simulink model "Vehicle_Model_2Track_r2018b"  (R2018b)
settings: Solver=FixedStepAuto  SolverName=FixedStepDiscrete  StartTime=T0  StopTime=Tf  FixedStep=Ts  EnableMultiTasking=on
model workspace (MAT data in the model file):
  aKalman = Simulink.Parameter
  aKalman.DataType = 'auto'
  aKalman.Dimensions = [0 0]
  slipEnabler = Simulink.Parameter
  slipEnabler.DataType = 'auto'
  slipEnabler.Dimensions = [0 0]
values from neighbouring files (symbols this model uses):
  longCTRparam = longitController()    [mainVehicleModel_2Track.m]
  pacejkaParam = loadPacejkaParam()    [mainVehicleModel_2Track.m]
  Ts = simulationPars.times.step_size    [mainVehicleModel_2Track.m]
  vehicle_data = getVehicleDataStruct()    [mainVehicleModel_2Track.m]
  X0 = loadInitialConditions    [mainVehicleModel_2Track.m]
undefined symbols (not defined in the file or in its folder): DiscIntNeverNeededParam
libraries: simulink_extras x11
settings Model: Creator=Edoardo  LastModifiedBy=tonegas
settings DataIOCC: LimitDataPoints=on  SaveFormat=Array  ReturnWorkspaceOutputs=on
settings OptimizationCC: DefaultParameterBehavior=Inlined  PassReuseOutputArgsAs=Individual arguments  MaxStackSize=64
settings DebuggingCC: ReadBeforeWriteMsg=DisableAll  WriteAfterWriteMsg=DisableAll  WriteAfterReadMsg=DisableAll  MultiTaskDSMMsg=none  ParameterTunabilityLossMsg=error  SFUnexpectedBacktrackingDiag=warning  SFNoUnconditionalDefaultTransitionDiag=warning  SFExecutionAtInitializationDiag=none
settings HardwareCC: ProdBitPerInt=16  ProdBitPerPointer=16  ProdBitPerSizeT=16  ProdBitPerPtrDiffT=16  ProdLargestAtomicFloat=None  ProdWordSize=16  ProdHWDeviceType=STMicroelectronics->ST10/Super10
settings ModelReferenceCC: UpdateModelReferenceTargets=IfOutOfDate  PropagateSignalLabelsOutOfModel=off
settings SFSimCC: SFSimEcho=off  SimUseLocalCustomCode=off  MATLABDynamicMemAlloc=off
settings RTWCC: SystemTargetFile=ert.tlc  TemplateMakefile=ert_default_tmf  GenerateReport=on  RetainRTWFile=on  RTWUseLocalCustomCode=off  Toolchain=GNU Tools for ARM Embedded Processors  BuildConfiguration=Faster Runs  IncludeHyperlinkInReport=on  LaunchReport=on  GenerateTraceInfo=on  GenerateTraceReport=on  GenerateTraceReportSl=on  GenerateTraceReportSf=on  GenerateTraceReportEml=on
settings CodeAppCC: ForceParamTrailComments=on  IgnoreCustomStorageClasses=off  OperatorAnnotations=on  SimulinkDataObjDesc=on  SFDataObjDesc=on  InsertBlockDesc=on
settings ERTTargetCC: CodeReplacementLibrary=ARM Cortex-M (Optimized)  SupportVariableSizeSignals=on  RootIOFormat=Structure reference  ERTCustomFileTemplate=example_file_process.tlc
settings ConfigComp: CovMetricSettings=dw  CovSaveCumulativeToWorkspaceVar=on  CovSaveSingleToWorkspaceVar=on  CovExternalEMLEnable=off

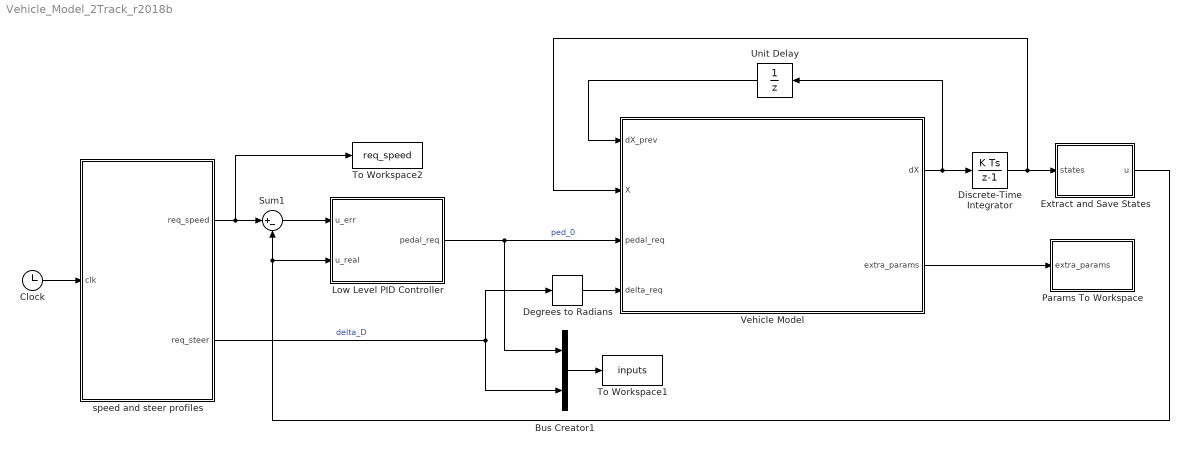
== system Vehicle_Model_2Track_r2018b ==
  Bus Creator1 : BusCreator  Inputs=2
  Clock : Clock
  Degrees to Radians : simulink_extras/Transformations/Degrees to Radians
  Discrete-Time Integrator : DiscreteIntegrator  gainval=1  InitialCondition=X0  SampleTime=-1  ICPrevOutput=DiscIntNeverNeededParam  ICPrevScaledInput=DiscIntNeverNeededParam
  Extract and Save States : Subsystem
  Low Level PID Controller : Subsystem
  Params To Workspace : Subsystem
  Sum1 : Sum  Inputs=|+-
  To Workspace1 : ToWorkspace  VariableName=inputs  SaveFormat=Timeseries  SampleTime=-1
  To Workspace2 : ToWorkspace  VariableName=req_speed  SaveFormat=Timeseries  SampleTime=-1
  Unit Delay : UnitDelay  InitialCondition=zeros(size(X0))  SampleTime=-1  HasFrameUpgradeWarning=on
  Vehicle Model : MATLAB Function  TreatAsAtomicUnit=on
  speed and steer profiles : MATLAB Function  TreatAsAtomicUnit=on
  wires:
  Vehicle Model/2(extra_params) -> Params To Workspace/1(extra_params)
  Discrete-Time Integrator/1 -> Extract and Save States/1(states), Vehicle Model/2(X)
  Vehicle Model/1(dX) -> Unit Delay/1, Discrete-Time Integrator/1
  Bus Creator1/1 -> To Workspace1/1
  speed and steer profiles/2(req_steer) -> Degrees to Radians/1, Bus Creator1/2  "delta_D"
  Degrees to Radians/1 -> Vehicle Model/4(delta_req)
  Clock/1 -> speed and steer profiles/1(clk)
  Low Level PID Controller/1(pedal_req) -> Vehicle Model/3(pedal_req), Bus Creator1/1  "ped_0"
  Unit Delay/1 -> Vehicle Model/1(dX_prev)
  Extract and Save States/1(u) -> Sum1/2, Low Level PID Controller/2(u_real)
  speed and steer profiles/1(req_speed) -> To Workspace2/1, Sum1/1
  Sum1/1 -> Low Level PID Controller/1(u_err)

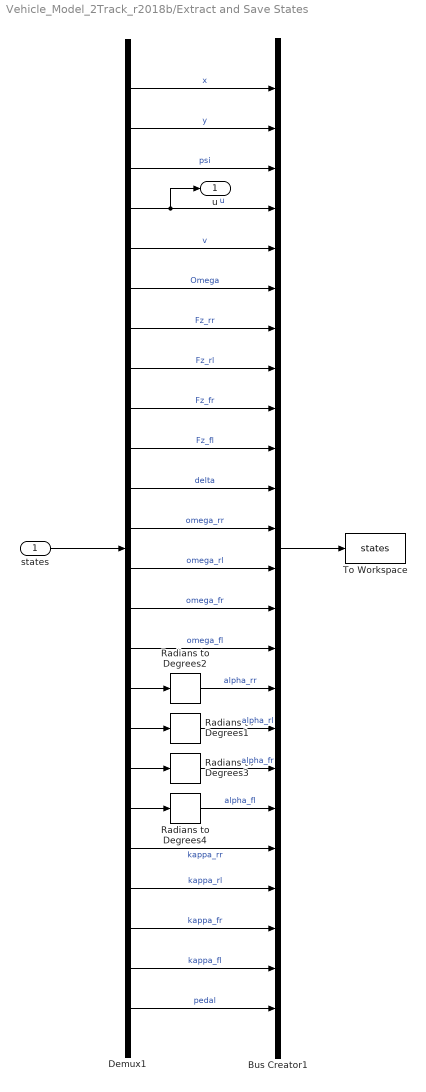
== system Vehicle_Model_2Track_r2018b/Extract and Save States ==
  states : Inport
  Bus Creator1 : BusCreator  Inputs=24
  Demux1 : Demux  Outputs=24
  Radians to Degrees{1..4} (4 alike) : simulink_extras/Transformations/Radians to Degrees
  To Workspace : ToWorkspace  VariableName=states  SaveFormat=Timeseries  SampleTime=-1
  u : Outport
  wires:
  Demux1/13 -> Bus Creator1/13  "omega_rl"
  Demux1/8 -> Bus Creator1/8  "Fz_rl"
  Demux1/23 -> Bus Creator1/23  "kappa_fl"
  Demux1/19 -> Radians to Degrees4/1
  states/1 -> Demux1/1
  Demux1/14 -> Bus Creator1/14  "omega_fr"
  Demux1/7 -> Bus Creator1/7  "Fz_rr"
  Demux1/15 -> Bus Creator1/15  "omega_fl"
  Demux1/3 -> Bus Creator1/3  "psi"
  Demux1/22 -> Bus Creator1/22  "kappa_fr"
  Demux1/4 -> u/1, Bus Creator1/4  "u"
  Demux1/6 -> Bus Creator1/6  "Omega"
  Demux1/11 -> Bus Creator1/11  "delta"
  Demux1/5 -> Bus Creator1/5  "v"
  Demux1/9 -> Bus Creator1/9  "Fz_fr"
  Demux1/21 -> Bus Creator1/21  "kappa_rl"
  Demux1/12 -> Bus Creator1/12  "omega_rr"
  Demux1/17 -> Radians to Degrees1/1
  Demux1/2 -> Bus Creator1/2  "y"
  Demux1/20 -> Bus Creator1/20  "kappa_rr"
  Demux1/10 -> Bus Creator1/10  "Fz_fl"
  Demux1/18 -> Radians to Degrees3/1
  Demux1/1 -> Bus Creator1/1  "x"
  Demux1/16 -> Radians to Degrees2/1
  Bus Creator1/1 -> To Workspace/1
  Radians to Degrees2/1 -> Bus Creator1/16  "alpha_rr"
  Radians to Degrees1/1 -> Bus Creator1/17  "alpha_rl"
  Radians to Degrees3/1 -> Bus Creator1/18  "alpha_fr"
  Radians to Degrees4/1 -> Bus Creator1/19  "alpha_fl"
  Demux1/24 -> Bus Creator1/24  "pedal"

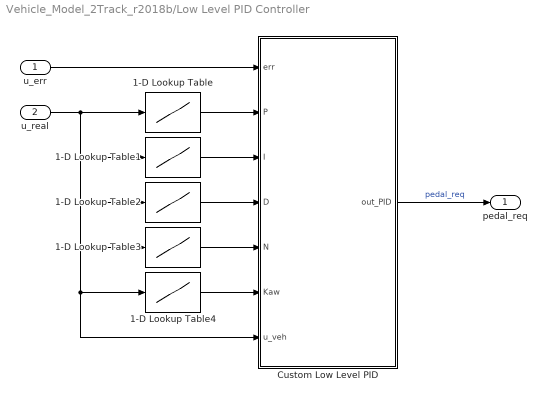
== system Vehicle_Model_2Track_r2018b/Low Level PID Controller ==
  u_err : Inport
  u_real : Inport  Port=2
  1-D Lookup Table : Lookup_n-D  NumberOfTableDimensions=1  BreakpointsForDimension1=longCTRparam.speed_vals_PID_sched  BeginIndexSearchUsingPreviousIndexResult=on  Table=longCTRparam.Kp_vals  ExtrapMethod=Clip  UseLastTableValue=on  InternalRulePriority=Speed  RndMeth=Simplest  InputSameDT=on
  1-D Lookup Table1 : Lookup_n-D  NumberOfTableDimensions=1  BreakpointsForDimension1=longCTRparam.speed_vals_PID_sched  BeginIndexSearchUsingPreviousIndexResult=on  Table=longCTRparam.Ki_vals  ExtrapMethod=Clip  UseLastTableValue=on  InternalRulePriority=Speed  RndMeth=Simplest  InputSameDT=on
  1-D Lookup Table2 : Lookup_n-D  NumberOfTableDimensions=1  BreakpointsForDimension1=longCTRparam.speed_vals_PID_sched  BeginIndexSearchUsingPreviousIndexResult=on  Table=longCTRparam.Kd_vals  ExtrapMethod=Clip  UseLastTableValue=on  InternalRulePriority=Speed  RndMeth=Simplest  InputSameDT=on
  1-D Lookup Table3 : Lookup_n-D  NumberOfTableDimensions=1  BreakpointsForDimension1=longCTRparam.speed_vals_PID_sched  BeginIndexSearchUsingPreviousIndexResult=on  Table=longCTRparam.N_vals  ExtrapMethod=Clip  UseLastTableValue=on  InternalRulePriority=Speed  RndMeth=Simplest  InputSameDT=on
  1-D Lookup Table4 : Lookup_n-D  NumberOfTableDimensions=1  BreakpointsForDimension1=longCTRparam.speed_vals_PID_sched  BeginIndexSearchUsingPreviousIndexResult=on  Table=longCTRparam.Kaw_vals  ExtrapMethod=Clip  UseLastTableValue=on  InternalRulePriority=Speed  RndMeth=Simplest  InputSameDT=on
  Custom Low Level PID : Subsystem
  pedal_req : Outport  VectorParamsAs1DForOutWhenUnconnected=off
  wires:
  1-D Lookup Table/1 -> Custom Low Level PID/2(P)
  u_err/1 -> Custom Low Level PID/1(err)
  u_real/1 -> 1-D Lookup Table4/1, Custom Low Level PID/7(u_veh), 1-D Lookup Table3/1, 1-D Lookup Table2/1, 1-D Lookup Table1/1, 1-D Lookup Table/1
  1-D Lookup Table2/1 -> Custom Low Level PID/4(D)
  1-D Lookup Table3/1 -> Custom Low Level PID/5(N)
  1-D Lookup Table1/1 -> Custom Low Level PID/3(I)
  Custom Low Level PID/1(out_PID) -> pedal_req/1  "pedal_req"
  1-D Lookup Table4/1 -> Custom Low Level PID/6(Kaw)

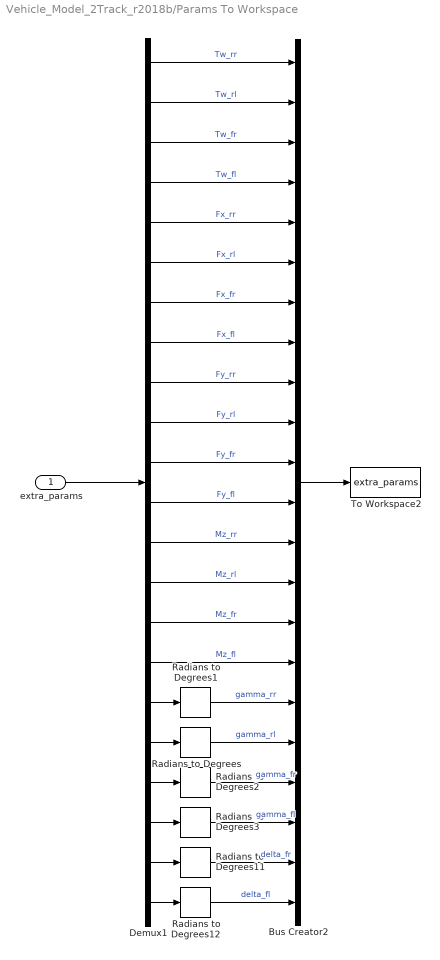
== system Vehicle_Model_2Track_r2018b/Params To Workspace ==
  extra_params : Inport
  Bus Creator2 : BusCreator  Inputs=22
  Demux1 : Demux  Outputs=22
  Radians to Degrees{,1..3,11..12} (6 alike) : simulink_extras/Transformations/Radians to Degrees
  To Workspace2 : ToWorkspace  VariableName=extra_params  SaveFormat=Timeseries  SampleTime=-1
  wires:
  Demux1/17 -> Radians to Degrees1/1
  Demux1/3 -> Bus Creator2/3  "Tw_fr"
  Radians to Degrees3/1 -> Bus Creator2/20  "gamma_fl"
  Demux1/16 -> Bus Creator2/16  "Mz_fl"
  Radians to Degrees1/1 -> Bus Creator2/17  "gamma_rr"
  Radians to Degrees11/1 -> Bus Creator2/21  "delta_fr"
  Demux1/14 -> Bus Creator2/14  "Mz_rl"
  Demux1/4 -> Bus Creator2/4  "Tw_fl"
  Demux1/6 -> Bus Creator2/6  "Fx_rl"
  Demux1/8 -> Bus Creator2/8  "Fx_fl"
  Demux1/13 -> Bus Creator2/13  "Mz_rr"
  Demux1/7 -> Bus Creator2/7  "Fx_fr"
  Demux1/5 -> Bus Creator2/5  "Fx_rr"
  Demux1/9 -> Bus Creator2/9  "Fy_rr"
  Demux1/11 -> Bus Creator2/11  "Fy_fr"
  Demux1/15 -> Bus Creator2/15  "Mz_fr"
  Demux1/10 -> Bus Creator2/10  "Fy_rl"
  Radians to Degrees12/1 -> Bus Creator2/22  "delta_fl"
  Radians to Degrees2/1 -> Bus Creator2/19  "gamma_fr"
  extra_params/1 -> Demux1/1
  Demux1/12 -> Bus Creator2/12  "Fy_fl"
  Bus Creator2/1 -> To Workspace2/1
  Demux1/1 -> Bus Creator2/1  "Tw_rr"
  Demux1/2 -> Bus Creator2/2  "Tw_rl"
  Radians to Degrees/1 -> Bus Creator2/18  "gamma_rl"
  Demux1/18 -> Radians to Degrees/1
  Demux1/19 -> Radians to Degrees2/1
  Demux1/20 -> Radians to Degrees3/1
  Demux1/21 -> Radians to Degrees11/1
  Demux1/22 -> Radians to Degrees12/1

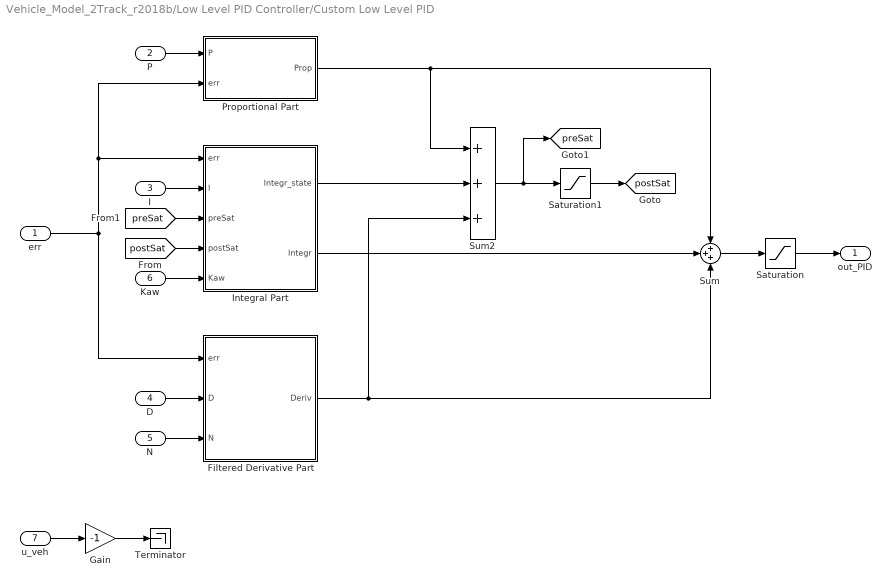
== system Vehicle_Model_2Track_r2018b/Low Level PID Controller/Custom Low Level PID ==
  err : Inport
  P : Inport  Port=2
  I : Inport  Port=3
  D : Inport  Port=4
  N : Inport  Port=5
  Kaw : Inport  Port=6
  u_veh : Inport  Port=7
  Filtered Derivative Part : Subsystem
  Gain : Gain  Gain=-1
  Integral Part : Subsystem
  Proportional Part : Subsystem
  Saturation : Saturate  UpperLimit=1  LowerLimit=-1  LinearizeAsGain=off
  Saturation1 : Saturate  UpperLimit=1  LowerLimit=-1  LinearizeAsGain=off
  Sum : Sum  Inputs=+++
  Sum2 : Sum  Inputs=+++
  Terminator : Terminator
  out_PID : Outport  VectorParamsAs1DForOutWhenUnconnected=off
  tag scope: postSat=global, preSat=global
  wires:
  Sum2/1 -> [preSat], Saturation1/1
  Sum/1 -> Saturation/1
  Saturation/1 -> out_PID/1
  err/1 -> Filtered Derivative Part/1(err), Proportional Part/2(err), Integral Part/1(err)
  Saturation1/1 -> [postSat]
  I/1 -> Integral Part/2(I)
  Integral Part/1(Integr_state) -> Sum2/2
  Integral Part/2(Integr) -> Sum/2
  Proportional Part/1(Prop) -> Sum2/1, Sum/1
  P/1 -> Proportional Part/1(P)
  [preSat] -> Integral Part/3(preSat)
  [postSat] -> Integral Part/4(postSat)
  Filtered Derivative Part/1(Deriv) -> Sum/3, Sum2/3
  D/1 -> Filtered Derivative Part/2(D)
  N/1 -> Filtered Derivative Part/3(N)
  u_veh/1 -> Gain/1
  Gain/1 -> Terminator/1
  Kaw/1 -> Integral Part/5(Kaw)

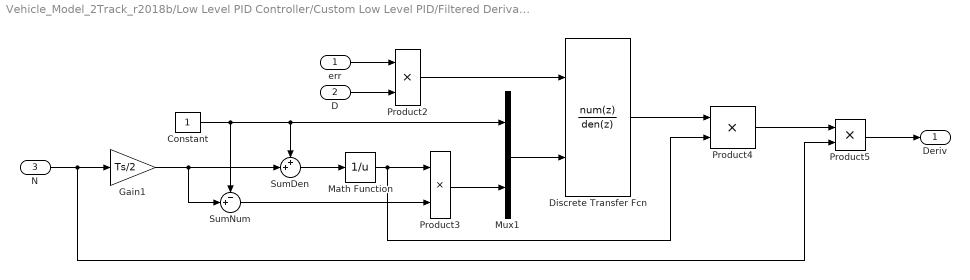
== system Vehicle_Model_2Track_r2018b/Low Level PID Controller/Custom Low Level PID/Filtered Derivative Part ==
  err : Inport
  D : Inport  Port=2
  N : Inport  Port=3
  Constant : Constant
  Discrete Transfer Fcn : DiscreteTransferFcn  Numerator=[1 -1]  DenominatorSource=Input port  SampleTime=Ts  a0EqualsOne=on
      settings: InputPortMap=u0,p3
  Gain1 : Gain  Gain=Ts/2
  Math Function : Math  Operator=reciprocal  SaturateOnIntegerOverflow=on
  Mux1 : Mux  Inputs=2
  Product{2..5} (4 alike) : Product
  SumDen : Sum  Inputs=++|
  SumNum : Sum  Inputs=-+|
  Deriv : Outport  VectorParamsAs1DForOutWhenUnconnected=off
  wires:
  N/1 -> Gain1/1, Product5/2
  Product4/1 -> Product5/1
  SumDen/1 -> Math Function/1
  Math Function/1 -> Product4/2, Product3/1
  SumNum/1 -> Product3/2
  Product2/1 -> Discrete Transfer Fcn/1
  Discrete Transfer Fcn/1 -> Product4/1
  Constant/1 -> SumNum/1, SumDen/1, Mux1/1
  Product3/1 -> Mux1/2
  Mux1/1 -> Discrete Transfer Fcn/2
  Gain1/1 -> SumNum/2, SumDen/2
  err/1 -> Product2/1
  D/1 -> Product2/2
  Product5/1 -> Deriv/1

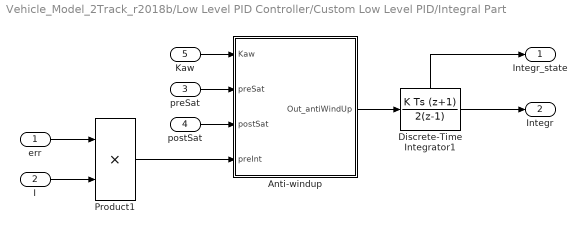
== system Vehicle_Model_2Track_r2018b/Low Level PID Controller/Custom Low Level PID/Integral Part ==
  err : Inport
  I : Inport  Port=2
  preSat : Inport  Port=3
  postSat : Inport  Port=4
  Kaw : Inport  Port=5
  Anti-windup : Subsystem
  Discrete-Time Integrator1 : DiscreteIntegrator  IntegratorMethod=Integration: Trapezoidal  SampleTime=Ts  ShowStatePort=on  ICPrevOutput=DiscIntNeverNeededParam  ICPrevScaledInput=DiscIntNeverNeededParam
  Product1 : Product
  Integr_state : Outport  VectorParamsAs1DForOutWhenUnconnected=off
  Integr : Outport  Port=2  VectorParamsAs1DForOutWhenUnconnected=off
  wires:
  Discrete-Time Integrator1/State -> Integr_state/1
  preSat/1 -> Anti-windup/2(preSat)
  Product1/1 -> Anti-windup/4(preInt)
  postSat/1 -> Anti-windup/3(postSat)
  I/1 -> Product1/2
  Anti-windup/1(Out_antiWindUp) -> Discrete-Time Integrator1/1
  Discrete-Time Integrator1/1 -> Integr/1
  err/1 -> Product1/1
  Kaw/1 -> Anti-windup/1(Kaw)

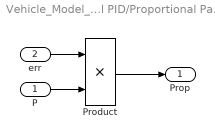
== system Vehicle_Model_2Track_r2018b/Low Level PID Controller/Custom Low Level PID/Proportional Part ==
  P : Inport
  err : Inport  Port=2
  Product : Product
  Prop : Outport  VectorParamsAs1DForOutWhenUnconnected=off
  wires:
  P/1 -> Product/2
  Product/1 -> Prop/1
  err/1 -> Product/1

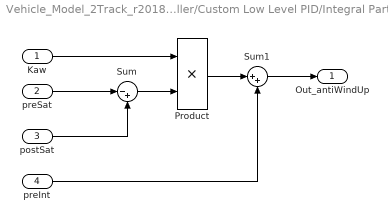
== system Vehicle_Model_2Track_r2018b/Low Level PID Controller/Custom Low Level PID/Integral Part/Anti-windup ==
  Kaw : Inport
  preSat : Inport  Port=2
  postSat : Inport  Port=3
  preInt : Inport  Port=4
  Product : Product
  Sum : Sum  Inputs=|-+
  Sum1 : Sum  Inputs=|++
  Out_antiWindUp : Outport  VectorParamsAs1DForOutWhenUnconnected=off
  wires:
  preSat/1 -> Sum/1
  preInt/1 -> Sum1/2
  Product/1 -> Sum1/1
  Sum1/1 -> Out_antiWindUp/1
  Sum/1 -> Product/2
  postSat/1 -> Sum/2
  Kaw/1 -> Product/1

== matlab function Vehicle_Model_2Track_r2018b/speed and steer profiles ==
  data: clk input; req_speed output; req_steer output
function [req_speed,req_steer] = speed_steer_profiles(clk)

    % ----------------------------------------------------------------
    %% Function purpose: compute the desired pedal and steer profiles
    % ----------------------------------------------------------------
    
    % Requested speed [m/s] for this time step
    req_speed = 100/3.6;  
    
    % Requested steering angle [deg] at the steering wheel for this time step
    req_steer = 12*sin(2*pi*0.018*clk);

end

== matlab function Vehicle_Model_2Track_r2018b/Vehicle Model ==
  settings: sampleTime=step_size
  data: dX_prev input; X input; dX output; extra_params output; pedal_req input; delta_req input; pacejkaParam parameter; vehicle_data parameter
function [dX,extra_params] = Vehicle_model(dX_prev,X,pedal_req,delta_req,pacejkaParam,vehicle_data)

    %% PASTE HERE YOUR VEHICLE MODEL

end
